simulink model "test_anarx_online"  (R2019a)
settings: Solver=FixedStepAuto  StartTime=0.0  StopTime=10.0  FixedStep=2.5e-4  RelTol=1e-3  EnableMultiTasking=on
PostLoadFcn:
  | , if any(exist('dsrtsu_mdlpostloadfcn', 'file') == [2, 3, 6]), try dsrtsu_mdlpostloadfcn('Execute', bdroot); catch fprintf('Error in PostLoadFcn (dsrtsu_mdlpostloadfcn) for model "%s":\n %s\n', bdroot, lasterr); end, end,
InitFcn:
  | Sicherheitssysteme_INIT
PreSaveFcn:
  | , if any(exist('dsmpb_private', 'file') == [2, 3, 6]), try, dsmpb_private('dsmpb_mdlclblib', 'PreSave', bdroot); catch, disp(lasterr); end, end,
CloseFcn:
  | , if any(exist('dsmpb_private', 'file') == [2, 3, 6]), try, dsmpb_private('dsmpb_mdlclblib', 'Close', bdroot); catch, disp(lasterr); end, end,
settings Model: DSMPB_DATASERVER_ModelPortLibVersion1=8  DSMPB_DATASERVER_DataServerVersion1=6  DSMPB_DATASERVER_DataServerStreamVersion1=3  Creator=CableRobot  LastModifiedBy=brandlju
settings SolverCC: AutoInsertRateTranBlk=on
settings DataIOCC: ReturnWorkspaceOutputs=off
settings OptimizationCC: LocalBlockOutputs=off
settings DebuggingCC: SFUnexpectedBacktrackingDiag=warning  SFNoUnconditionalDefaultTransitionDiag=warning  ArithmeticOperatorsInVariantConditions=warning
settings SFSimCC: SimUseLocalCustomCode=off
settings RTWCC: SystemTargetFile=TwinCAT.tlc  GenCodeOnly=on  MakeCommand=make_tct  TemplateMakefile=tct_msbuild.tmf  Description=TwinCAT Target  GenerateReport=on  RTWUseLocalCustomCode=off  TargetLang=C++
settings CodeAppCC: StateflowObjectComments=on
settings STFCustomTargetCC: TargetLangStandard=C++03 (ISO)  CompOptLevelCompliant=on  MATLABClassNameForMDSCustomization=Simulink.SoftwareTarget.TargetSpecificTriggerConfigurationBase  SystemTargetFile=TwinCAT.tlc
settings ConfigComp: CovMetricSettings=dw  CovHtmlReporting=on  CovSaveCumulativeToWorkspaceVar=on  CovSaveSingleToWorkspaceVar=on  CovExternalEMLEnable=off

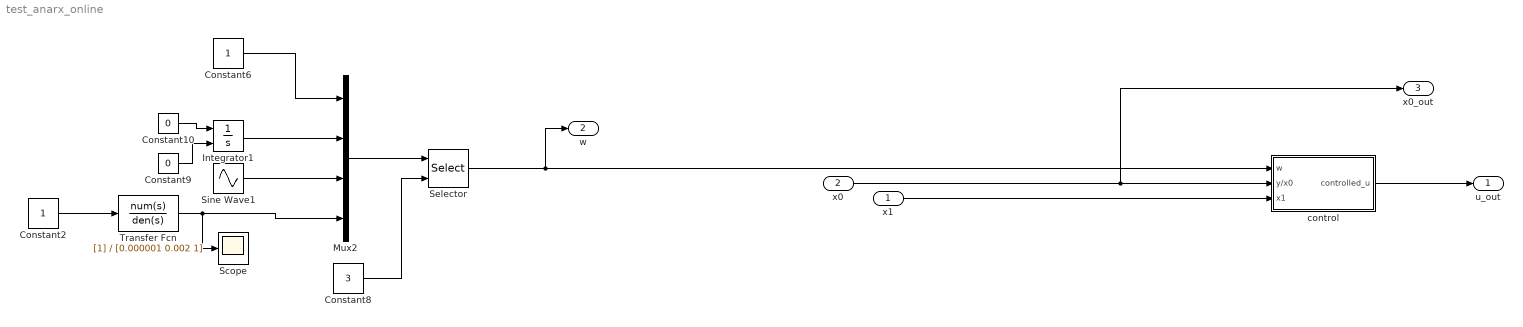
== system test_anarx_online ==
  x1 : Inport  OutDataTypeStr=double  PortDimensions=1
  x0 : Inport  Port=2
  Constant10 : Constant  Value=0
  Constant2 : Constant
  Constant6 : Constant
  Constant8 : Constant  Value=3
  Constant9 : Constant  Value=0
  Integrator1 : Integrator  ExternalReset=either
  Mux2 : Mux
  Scope : Scope
  Selector : Selector  InputPortWidth=4  IndexOptions=Index vector (port)  Indices=[1 3]  OutputSizes=1
  Sine Wave1 : Sin  Frequency=0.1  SampleTime=0
  Transfer Fcn : TransferFcn  Denominator=[0.000001 0.002 1]
  control : Subsystem
  u_out : Outport
  w : Outport  Port=2
  x0_out : Outport  Port=3
  wires:
  Constant10/1 -> Integrator1/1
  Constant9/1 -> Integrator1/2
  Constant8/1 -> Selector/2
  Sine Wave1/1 -> Mux2/3
  Integrator1/1 -> Mux2/2
  Constant6/1 -> Mux2/1
  Mux2/1 -> Selector/1
  x1/1 -> control/3(x1)
  Selector/1 -> w/1, control/1(w)
  Constant2/1 -> Transfer Fcn/1
  Transfer Fcn/1 -> Scope/1, Mux2/4
  control/1(controlled_u) -> u_out/1
  x0/1 -> x0_out/1, control/2(y/x0)

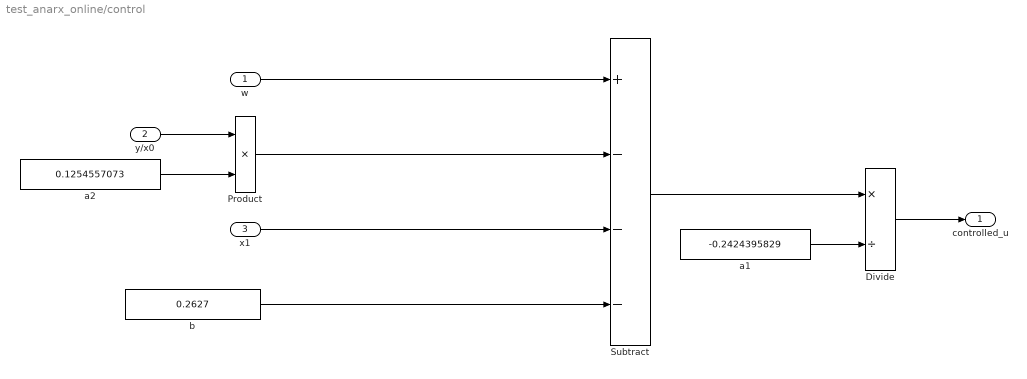
== system test_anarx_online/control ==
  w : Inport
  y/x0 : Inport  Port=2
  x1 : Inport  Port=3
  Divide : Product  Inputs=*/
  Product : Product
  Subtract : Sum  Inputs=+---
  a1 : Constant  Value=-0.2424395829
  a2 : Constant  Value=0.1254557073
  b : Constant  Value=0.2627
  controlled_u : Outport  VectorParamsAs1DForOutWhenUnconnected=on
  wires:
  y/x0/1 -> Product/1
  a2/1 -> Product/2
  w/1 -> Subtract/1
  Product/1 -> Subtract/2
  x1/1 -> Subtract/3
  b/1 -> Subtract/4
  Subtract/1 -> Divide/1
  a1/1 -> Divide/2
  Divide/1 -> controlled_u/1
